simulink model "EV_PV_Charging"  (R2025a)
settings: Solver=ode3  StartTime=0.0  StopTime=1  RelTol=1e-3
PreLoadFcn:
  | %% Parameter file: OBC_4_data.m
  | 
  | %% Model Parameters
  | Ts_Power= 50e-9;        % SPS Model sample time (s)
  | Co=150e-6;              % Output filter (F)
  | Ron_FET=50e-3;          % FET resistance (ohms)
  | Ron_Diode=50e-3;        % FET resistance (ohms)
  | Vf=0.6;                 % Diode forward voltage (V)
  | %
  | %% PFC Data
  | Vnom_ac= 240;           % Nominal Ac voltage (V)
  | Fnom= 60;               % System frequency (Hz)
  | L_PFC= 600e-6;          % PFC Inductance (H)
  | RL_PFC= 20e-3;          % Inductance resistance (Ohm)
  | C_PFC= 2600e-6;         % Capacitance (F)
  | 
  | %% PFC Control System Parameters
  | Ts_Control= 10e-6;      % Control system time (s)
  | Fsw= 100e3;             % PWM Switching frequency (Hz)
  | DT_PFC=400e-9;
  | %
  | % Current Regulator (PR):
  | Kp_I= 0.06;             % Proportional gain
  | Kr_I= 2.5;              % Resonant gain
  | Zeta_I=0.2;             % Damping coefficient
  | Fr_I=Fnom*2;            % Resonant frequency (Hz)
  | %
  | % Voltage Regulator (PI):
  | Kp_V= 0.25;             % Proportional gain
  | Ki_V= 80;               % Integral gain
  | Limit_V= 100;           % Output limit
  | %
  | %% LLC Data
  | Vdc_in=400;             % DC input voltage (V)
  | Vo_nom=400;             % DC nominal output voltage (V)
  | Po_nom=7.2e3;           % Nominal output power (W)
  | Lr=25e-6;               % Transformer leakage inductance (Resonant inductance in Henry)
  | Lm=150e-6;              % Magnetization inductance (H)
  | Cr=75e-9;               % Resonant capacitor (F)
  | Np=10; Ns=12; N=Np/Ns;  % Transformer ratio
  | %
  | %% LLC Control System Parameters
  | DT_LLC=400e-9;
  | Ts_Control=10e-6;
  | % Voltage Regulator (PI):
  | Kp_LLC= 100/4;          % Proportional gain
  | Ki_LLC= 150e3;          % Integral gain
  | fs_LCC_min= 120e3;      % Minimum switching frequency (Hz)
  | fs_LCC_max= 300e3;      % Maximum switching frequency (Hz)
  | Vref_LCC_min= 275;      % Minimum voltage setpoint (V)
  | Vref_LCC_max= 450;      % Maximum voltage setpoint (V)
  | %
  | %%
  | % Resonant tank data
  | Ro=Vo_nom^2/Po_nom      % LLC output load (Ohm)
  | Rac=(8/pi^2)*N^2*Ro     % Equivalent pprimary AC resistance (Ohm)
  | Q=sqrt(Lr/Cr)/Rac       % Quality factor
  | fr=1/(2*pi*sqrt(Lr*Cr)) % Resonant frequency (Hz)
  | m=(Lr+Lm)/Lr            % Ratio of total primary reactance to resonant inductance (Lr)
  | %%
InitFcn:
  | %% Parameter file: OBC_4_data.m
  | 
  | %% Model Parameters
  | Ts_Power= 50e-9;        % SPS Model sample time (s)
  | Co=150e-6;              % Output filter (F)
  | Ron_FET=50e-3;          % FET resistance (ohms)
  | Ron_Diode=50e-3;        % FET resistance (ohms)
  | Vf=0.6;                 % Diode forward voltage (V)
  | %
  | %% PFC Data
  | Vnom_ac= 240;           % Nominal Ac voltage (V)
  | Fnom= 60;               % System frequency (Hz)
  | L_PFC= 600e-6;          % PFC Inductance (H)
  | RL_PFC= 20e-3;          % Inductance resistance (Ohm)
  | C_PFC= 2600e-6;         % Capacitance (F)
  | 
  | %% PFC Control System Parameters
  | Ts_Control= 10e-6;      % Control system time (s)
  | Fsw= 100e3;             % PWM Switching frequency (Hz)
  | DT_PFC=400e-9;
  | %
  | % Current Regulator (PR):
  | Kp_I= 0.06;             % Proportional gain
  | Kr_I= 2.5;              % Resonant gain
  | Zeta_I=0.2;             % Damping coefficient
  | Fr_I=Fnom*2;            % Resonant frequency (Hz)
  | %
  | % Voltage Regulator (PI):
  | Kp_V= 0.25;             % Proportional gain
  | Ki_V= 80;               % Integral gain
  | Limit_V= 100;           % Output limit
  | %
  | %% LLC Data
  | Vdc_in=400;             % DC input voltage (V)
  | Vo_nom=400;             % DC nominal output voltage (V)
  | Po_nom=7.2e3;           % Nominal output power (W)
  | Lr=25e-6;               % Transformer leakage inductance (Resonant inductance in Henry)
  | Lm=150e-6;              % Magnetization inductance (H)
  | Cr=75e-9;               % Resonant capacitor (F)
  | Np=10; Ns=12; N=Np/Ns;  % Transformer ratio
  | %
  | %% LLC Control System Parameters
  | DT_LLC=400e-9;
  | Ts_Control=10e-6;
  | % Voltage Regulator (PI):
  | Kp_LLC= 100/4;          % Proportional gain
  | Ki_LLC= 150e3;          % Integral gain
  | fs_LCC_min= 120e3;      % Minimum switching frequency (Hz)
  | fs_LCC_max= 300e3;      % Maximum switching frequency (Hz)
  | Vref_LCC_min= 275;      % Minimum voltage setpoint (V)
  | Vref_LCC_max= 450;      % Maximum voltage setpoint (V)
  | %
  | %%
  | % Resonant tank data
  | Ro=Vo_nom^2/Po_nom      % LLC output load (Ohm)
  | Rac=(8/pi^2)*N^2*Ro     % Equivalent pprimary AC resistance (Ohm)
  | Q=sqrt(Lr/Cr)/Rac       % Quality factor
  | fr=1/(2*pi*sqrt(Lr*Cr)) % Resonant frequency (Hz)
  | m=(Lr+Lm)/Lr            % Ratio of total primary reactance to resonant inductance (Lr)
  | %%
undefined symbols (not defined in the file or in its folder): D1, Delta, DiscIntNeverNeededParam
libraries: spsSeriesRLCBranchLib x11, spsDiodeLib x7, spsMeanLib x6, MyLibrary x6, spsCurrentMeasurementLib x5, spsVoltageMeasurementLib x5, spsFourierLib x4, spsThreePhaseTransformerTwoWindingsLib x3, spsOnDelayLib x3, spsDistributedParametersLineLib x2, spsThreePhaseParallelRLCLoadLib x2, spsPWMGeneratorDCDCLib x2
(part 2 of 4)

== system EV_PV_Charging/600V Utlity Grid ==
  120 kV / 25 kV 47 MVA : spsThreePhaseTransformerTwoWindingsLib/Three-Phase Transformer (Two Windings)  Winding1Connection=Yg  Winding2Connection=Delta (D1)  CoreType=Three single-phase transformers  SetSaturation=off  Hysteresis=off  DataFile='basic_model'  SetInitialFlux=off  Measurements=None  UNITS=pu  NominalPower=[47e6 60 ]  Winding1="[ 120e3  0.08/30   0.08 ]"  Winding2="[ 25e3  0.08/30  0.08]"  Rm=500  Lm=500  L0=0.5  Saturation="[ 0,0  ;  0.005,1.2  ;  1.0,1.4 ]"  InitialFluxes=[ 0.8 , -0.8 , 0.7 ]  BreakLoop=off  DiscreteSolver=Trapezoidal iterative  DataType=off  TransfoNumber=0
  120kV 2500MVA : spsThreePhaseSourceLib/Three-Phase Source  InternalConnection=Yg  VoltagePhases=off  Voltage=120e3  PhaseAngle=0  Voltage_phases=[25e3 25e3 25e3]/sqrt(3)  PhaseAngles_phases=[0 -120 +120]  Frequency=60  NonIdealSource=on  SpecifyImpedance=on  Resistance=0.8929  Inductance=16.58e-3  ShortCircuitLevel=2500e6  BaseVoltage=120e3  XRratio=7  BusType=swing  Pref=0  Qref=0  Prefabc=[10e3, 10e3, 10e3]  Qrefabc=[0, 0, 0]  Qmin=-inf  Qmax=inf
  14-km Feeder : spsDistributedParametersLineLib/Distributed Parameters Line  Phases=3  Length=14  Frequency=60  Resistance=[0.1153 0.413]  Inductance=[1.05e-3 3.32e-3]  Capacitance=[11.33e-009 5.01e-009]  x1=[-5.71e-05 -1.91453846184522e-09 0 0;-5.705e-05 -1.91458738877014e-09 0 0;-5.7e-05 -1.9146363150148e-09 0 0;-5.695e-05 -1.91468524057917e-09 0 0;-5.69e-05 -1.91473416546325e-09 0 0;-5.685e-05 -1.91478308966701e-09 0 0;-5.68e-05 -1.91483201319044e-09 0 0;-5.675e-05 -1.91488093603352e-09 0 0;-5.67e-05 -1.91492985819623e-09 0 0;-5.665e-05 -1.91497877967855e-09 0 0;-5.66e-05 -1.91502770048047e-09 0 0;-5.655e-05 -1.91507662060197e-09 0 0;-5.65e-05 -1.91512554004303e-09 0 0;-5.645e-05 -1.91517445880364e-09 0 0;-5.64e-05 -1.91522337688377e-09 0 0;-5.635e-05 -1.91527229428342e-09 0 0;-5.63e-05 -1.91532121100256e-09 0 0;-5.625e-05 -1.91537012704117e-09 0 0;-5.62e-05 -1.91541904239924e-09 0 0;-5.615e-05 -1.91546795707675e-09 0 0;-5.61e-05 -1.91551687107368e-09 0 0;-5.605e-05 -1.91556578439002e-09 0 0;-5.6e-05 -1.91561469702575e-09 0 0;-5.595e-05 -1.91566360898085e-09 0 0;-5.59e-05 -1.91571252025531e-09 0 0;-5.585e-05 -1.9157614308491e-09 0 0;-5.58e-05 -1.9158103407622e-09 0 0;-5.575e-05 -1.91585924999461e-09 0 0;-5.57e-05 -1.91590815854631e-09 0 0;-5.565e-05 -1.91595706641727e-09 0 0;-5.56e-05 -1.91600597360748e-09 0 0;-5.555e-05 -1.91605488011692e-09 0 0;-5.55e-05 -1.91610378594558e-09 0 0;-5.545e-05 -1.91615269109344e-09 0 0;-5.54e-05 -1.91620159556047e-09 0 0;-5.535e-05 -1.91625049934667e-09 0 0;-5.53e-05 -1.91629940245201e-09 0 0;-5.525e-05 -1.91634830487648e-09 0 0;-5.52e-05 -1.91639720662006e-09 0 0;-5.515e-05 -1.91644610768273e-09 0 0;-5.51e-05 -1.91649500806448e-09 0 0;-5.505e-05 -1.91654390776529e-09 0 0;-5.5e-05 -1.91659280678514e-09 0 0;-5.495e-05 -1.91664170512401e-09 0 0;-5.49e-05 -1.91669060278189e-09 0 0;-5.485e-05 -1.91673949975876e-09 0 0;-5.48e-05 -1.91678839605459e-09 0 0;-5.475e-05 -1.91683729166939e-09 0 0;-5.47e-05 -1.91688618660312e-09 0 0;-5.465e-05 -1.91693508085576e-09 0 0;-5.46e-05 -1.91698397442731e-09 0 0;-5.455e-05 -1.91703286731775e-09 0 0;-5.45e-05 -1.91708175952705e-09 0 0;-5.445e-05 -1.9171306510552e-09 0 0;-5.44e-05 -1.91717954190219e-09 0 0;-5.435e-05 -1.91722843206799e-09 0 0;-5.43e-05 -1.91727732155258e-09 0 0;-5.425e-05 -1.91732621035596e-09 0 0;-5.42e-05 -1.9173750984781e-09 0 0;-5.415e-05 -1.91742398591899e-09 0 0;-5.41e-05 -1.9174728726786e-09 0 0;-5.405e-05 -1.91752175875693e-09 0 0;-5.4e-05 -1.91757064415394e-09 0 0;-5.395e-05 -1.91761952886964e-09 0 0;-5.39e-05 -1.91766841290399e-09 0 0;-5.385e-05 -1.91771729625699e-09 0 0;-5.38e-05 -1.91776617892861e-09 0 0;-5.375e-05 -1.91781506091883e-09 0 0;-5.37e-05 -1.91786394222765e-09 0 0;-5.365e-05 -1.91791282285503e-09 0 0;-5.36e-05 -1.91796170280097e-09 0 0;-5.355e-05 -1.91801058206545e-09 0 0;-5.35e-05 -1.91805946064845e-09 0 0;-5.345e-05 -1.91810833854995e-09 0 0;-5.34e-05 -1.91815721576993e-09 0 0;-5.335e-05 -1.91820609230839e-09 0 0;-5.33e-05 -1.91825496816529e-09 0 0;-5.325e-05 -1.91830384334063e-09 0 0;-5.32e-05 -1.91835271783438e-09 0 0;-5.315e-05 -1.91840159164653e-09 0 0;-5.31e-05 -1.91845046477706e-09 0 0;-5.305e-05 -1.91849933722596e-09 0 0;-5.3e-05 -1.9185482089932e-09 0 0;-5.295e-05 -1.91859708007877e-09 0 0;-5.29e-05 -1.91864595048265e-09 0 0;-5.285e-05 -1.91869482020482e-09 0 0;-5.28e-05 -1.91874368924527e-09 0 0;-5.275e-05 -1.91879255760398e-09 0 0;-5.27e-05 -1.91884142528094e-09 0 0;-5.265e-05 -1.91889029227611e-09 0 0;-5.26e-05 -1.9189391585895e-09 0 0;-5.255e-05 -1.91898802422107e-09 0 0;-5.25e-05 -1.91903688917082e-09 0 0;-5.245e-05 -1.91908575343872e-09 0 0;-5.24e-05 -1.91913461702476e-09 0 0;-5.235e-05 -1.91918347992892e-09 0 0;-5.23e-05 -1.91923234215119e-09 0 0;-5.225e-05 -1.91928120369154e-09 0 0;-5.22e-05 -1.91933006454995e-09 0 0;-5.215e-05 -1.91937892472642e-09 0 0;-5.21e-05 -1.91942778422092e-09 0 0;-5.205e-05 -1.91947664303344e-09 0 0;-5.2e-05 -1.91952550116396e-09 0 0;-5.195e-05 -1.91957435861246e-09 0 0;-5.19e-05 -1.91962321537892e-09 0 0;-5.185e-05 -1.91967207146333e-09 0 0;-5.18e-05 -1.91972092686567e-09 0 0;-5.175e-05 -1.91976978158592e-09 0 0;-5.17e-05 -1.91981863562407e-09 0 0;-5.165e-05 -1.91986748898009e-09 0 ...(+67941 chars)]  x2=[-5.71e-05 -2.09426061623554e-09 0 0;-5.705e-05 -2.09430829998972e-09 0 0;-5.7e-05 -2.09435598299977e-09 0 0;-5.695e-05 -2.09440366526568e-09 0 0;-5.69e-05 -2.09445134678745e-09 0 0;-5.685e-05 -2.09449902756504e-09 0 0;-5.68e-05 -2.09454670759844e-09 0 0;-5.675e-05 -2.09459438688764e-09 0 0;-5.67e-05 -2.09464206543262e-09 0 0;-5.665e-05 -2.09468974323336e-09 0 0;-5.66e-05 -2.09473742028984e-09 0 0;-5.655e-05 -2.09478509660205e-09 0 0;-5.65e-05 -2.09483277216998e-09 0 0;-5.645e-05 -2.09488044699359e-09 0 0;-5.64e-05 -2.09492812107289e-09 0 0;-5.635e-05 -2.09497579440784e-09 0 0;-5.63e-05 -2.09502346699844e-09 0 0;-5.625e-05 -2.09507113884466e-09 0 0;-5.62e-05 -2.09511880994649e-09 0 0;-5.615e-05 -2.09516648030391e-09 0 0;-5.61e-05 -2.09521414991691e-09 0 0;-5.605e-05 -2.09526181878547e-09 0 0;-5.6e-05 -2.09530948690957e-09 0 0;-5.595e-05 -2.09535715428919e-09 0 0;-5.59e-05 -2.09540482092432e-09 0 0;-5.585e-05 -2.09545248681495e-09 0 0;-5.58e-05 -2.09550015196104e-09 0 0;-5.575e-05 -2.09554781636259e-09 0 0;-5.57e-05 -2.09559548001959e-09 0 0;-5.565e-05 -2.095643142932e-09 0 0;-5.56e-05 -2.09569080509982e-09 0 0;-5.555e-05 -2.09573846652303e-09 0 0;-5.55e-05 -2.09578612720161e-09 0 0;-5.545e-05 -2.09583378713555e-09 0 0;-5.54e-05 -2.09588144632482e-09 0 0;-5.535e-05 -2.09592910476942e-09 0 0;-5.53e-05 -2.09597676246932e-09 0 0;-5.525e-05 -2.09602441942451e-09 0 0;-5.52e-05 -2.09607207563497e-09 0 0;-5.515e-05 -2.09611973110068e-09 0 0;-5.51e-05 -2.09616738582163e-09 0 0;-5.505e-05 -2.09621503979779e-09 0 0;-5.5e-05 -2.09626269302917e-09 0 0;-5.495e-05 -2.09631034551572e-09 0 0;-5.49e-05 -2.09635799725745e-09 0 0;-5.485e-05 -2.09640564825433e-09 0 0;-5.48e-05 -2.09645329850634e-09 0 0;-5.475e-05 -2.09650094801347e-09 0 0;-5.47e-05 -2.0965485967757e-09 0 0;-5.465e-05 -2.09659624479302e-09 0 0;-5.46e-05 -2.0966438920654e-09 0 0;-5.455e-05 -2.09669153859283e-09 0 0;-5.45e-05 -2.0967391843753e-09 0 0;-5.445e-05 -2.09678682941278e-09 0 0;-5.44e-05 -2.09683447370527e-09 0 0;-5.435e-05 -2.09688211725273e-09 0 0;-5.43e-05 -2.09692976005516e-09 0 0;-5.425e-05 -2.09697740211254e-09 0 0;-5.42e-05 -2.09702504342485e-09 0 0;-5.415e-05 -2.09707268399208e-09 0 0;-5.41e-05 -2.09712032381421e-09 0 0;-5.405e-05 -2.09716796289121e-09 0 0;-5.4e-05 -2.09721560122308e-09 0 0;-5.395e-05 -2.0972632388098e-09 0 0;-5.39e-05 -2.09731087565135e-09 0 0;-5.385e-05 -2.09735851174771e-09 0 0;-5.38e-05 -2.09740614709887e-09 0 0;-5.375e-05 -2.0974537817048e-09 0 0;-5.37e-05 -2.0975014155655e-09 0 0;-5.365e-05 -2.09754904868095e-09 0 0;-5.36e-05 -2.09759668105112e-09 0 0;-5.355e-05 -2.09764431267601e-09 0 0;-5.35e-05 -2.09769194355559e-09 0 0;-5.345e-05 -2.09773957368985e-09 0 0;-5.34e-05 -2.09778720307877e-09 0 0;-5.335e-05 -2.09783483172233e-09 0 0;-5.33e-05 -2.09788245962052e-09 0 0;-5.325e-05 -2.09793008677332e-09 0 0;-5.32e-05 -2.09797771318072e-09 0 0;-5.315e-05 -2.09802533884269e-09 0 0;-5.31e-05 -2.09807296375922e-09 0 0;-5.305e-05 -2.09812058793029e-09 0 0;-5.3e-05 -2.09816821135589e-09 0 0;-5.295e-05 -2.098215834036e-09 0 0;-5.29e-05 -2.0982634559706e-09 0 0;-5.285e-05 -2.09831107715967e-09 0 0;-5.28e-05 -2.0983586976032e-09 0 0;-5.275e-05 -2.09840631730118e-09 0 0;-5.27e-05 -2.09845393625358e-09 0 0;-5.265e-05 -2.09850155446038e-09 0 0;-5.26e-05 -2.09854917192158e-09 0 0;-5.255e-05 -2.09859678863714e-09 0 0;-5.25e-05 -2.09864440460707e-09 0 0;-5.245e-05 -2.09869201983133e-09 0 0;-5.24e-05 -2.09873963430992e-09 0 0;-5.235e-05 -2.09878724804281e-09 0 0;-5.23e-05 -2.09883486103e-09 0 0;-5.225e-05 -2.09888247327145e-09 0 0;-5.22e-05 -2.09893008476716e-09 0 0;-5.215e-05 -2.0989776955171e-09 0 0;-5.21e-05 -2.09902530552127e-09 0 0;-5.205e-05 -2.09907291477964e-09 0 0;-5.2e-05 -2.0991205232922e-09 0 0;-5.195e-05 -2.09916813105893e-09 0 0;-5.19e-05 -2.09921573807982e-09 0 0;-5.185e-05 -2.09926334435484e-09 0 0;-5.18e-05 -2.09931094988398e-09 0 0;-5.175e-05 -2.09935855466722e-09 0 0;-5.17e-05 -2.09940615870455e-09 0 0;-5.165e-05 -2.09945376199594e-09 0 0 ...(+67971 chars)]  x3=[-5.71e-05 -8.597316094106e-12 0 0;-5.705e-05 -8.59751457746718e-12 0 0;-5.7e-05 -8.59771305777361e-12 0 0;-5.695e-05 -8.59791153502522e-12 0 0;-5.69e-05 -8.59811000922194e-12 0 0;-5.685e-05 -8.59830848036371e-12 0 0;-5.68e-05 -8.59850694845045e-12 0 0;-5.675e-05 -8.59870541348209e-12 0 0;-5.67e-05 -8.59890387545856e-12 0 0;-5.665e-05 -8.59910233437979e-12 0 0;-5.66e-05 -8.59930079024571e-12 0 0;-5.655e-05 -8.59949924305624e-12 0 0;-5.65e-05 -8.59969769281133e-12 0 0;-5.645e-05 -8.59989613951089e-12 0 0;-5.64e-05 -8.60009458315487e-12 0 0;-5.635e-05 -8.60029302374318e-12 0 0;-5.63e-05 -8.60049146127575e-12 0 0;-5.625e-05 -8.60068989575252e-12 0 0;-5.62e-05 -8.60088832717341e-12 0 0;-5.615e-05 -8.60108675553837e-12 0 0;-5.61e-05 -8.6012851808473e-12 0 0;-5.605e-05 -8.60148360310015e-12 0 0;-5.6e-05 -8.60168202229684e-12 0 0;-5.595e-05 -8.60188043843731e-12 0 0;-5.59e-05 -8.60207885152148e-12 0 0;-5.585e-05 -8.60227726154928e-12 0 0;-5.58e-05 -8.60247566852064e-12 0 0;-5.575e-05 -8.60267407243549e-12 0 0;-5.57e-05 -8.60287247329376e-12 0 0;-5.565e-05 -8.60307087109538e-12 0 0;-5.56e-05 -8.60326926584028e-12 0 0;-5.555e-05 -8.60346765752839e-12 0 0;-5.55e-05 -8.60366604615964e-12 0 0;-5.545e-05 -8.60386443173396e-12 0 0;-5.54e-05 -8.60406281425127e-12 0 0;-5.535e-05 -8.60426119371152e-12 0 0;-5.53e-05 -8.60445957011461e-12 0 0;-5.525e-05 -8.60465794346049e-12 0 0;-5.52e-05 -8.60485631374909e-12 0 0;-5.515e-05 -8.60505468098034e-12 0 0;-5.51e-05 -8.60525304515416e-12 0 0;-5.505e-05 -8.60545140627048e-12 0 0;-5.5e-05 -8.60564976432923e-12 0 0;-5.495e-05 -8.60584811933035e-12 0 0;-5.49e-05 -8.60604647127377e-12 0 0;-5.485e-05 -8.6062448201594e-12 0 0;-5.48e-05 -8.60644316598719e-12 0 0;-5.475e-05 -8.60664150875705e-12 0 0;-5.47e-05 -8.60683984846893e-12 0 0;-5.465e-05 -8.60703818512275e-12 0 0;-5.46e-05 -8.60723651871843e-12 0 0;-5.455e-05 -8.60743484925592e-12 0 0;-5.45e-05 -8.60763317673514e-12 0 0;-5.445e-05 -8.60783150115601e-12 0 0;-5.44e-05 -8.60802982251847e-12 0 0;-5.435e-05 -8.60822814082245e-12 0 0;-5.43e-05 -8.60842645606788e-12 0 0;-5.425e-05 -8.60862476825468e-12 0 0;-5.42e-05 -8.60882307738279e-12 0 0;-5.415e-05 -8.60902138345213e-12 0 0;-5.41e-05 -8.60921968646264e-12 0 0;-5.405e-05 -8.60941798641425e-12 0 0;-5.4e-05 -8.60961628330688e-12 0 0;-5.395e-05 -8.60981457714046e-12 0 0;-5.39e-05 -8.61001286791492e-12 0 0;-5.385e-05 -8.6102111556302e-12 0 0;-5.38e-05 -8.61040944028622e-12 0 0;-5.375e-05 -8.61060772188291e-12 0 0;-5.37e-05 -8.61080600042021e-12 0 0;-5.365e-05 -8.61100427589803e-12 0 0;-5.36e-05 -8.61120254831632e-12 0 0;-5.355e-05 -8.61140081767499e-12 0 0;-5.35e-05 -8.61159908397399e-12 0 0;-5.345e-05 -8.61179734721323e-12 0 0;-5.34e-05 -8.61199560739266e-12 0 0;-5.335e-05 -8.61219386451219e-12 0 0;-5.33e-05 -8.61239211857176e-12 0 0;-5.325e-05 -8.6125903695713e-12 0 0;-5.32e-05 -8.61278861751073e-12 0 0;-5.315e-05 -8.61298686238999e-12 0 0;-5.31e-05 -8.61318510420901e-12 0 0;-5.305e-05 -8.61338334296771e-12 0 0;-5.3e-05 -8.61358157866603e-12 0 0;-5.295e-05 -8.6137798113039e-12 0 0;-5.29e-05 -8.61397804088123e-12 0 0;-5.285e-05 -8.61417626739797e-12 0 0;-5.28e-05 -8.61437449085405e-12 0 0;-5.275e-05 -8.61457271124939e-12 0 0;-5.27e-05 -8.61477092858392e-12 0 0;-5.265e-05 -8.61496914285757e-12 0 0;-5.26e-05 -8.61516735407028e-12 0 0;-5.255e-05 -8.61536556222196e-12 0 0;-5.25e-05 -8.61556376731256e-12 0 0;-5.245e-05 -8.615761969342e-12 0 0;-5.24e-05 -8.61596016831021e-12 0 0;-5.235e-05 -8.61615836421711e-12 0 0;-5.23e-05 -8.61635655706265e-12 0 0;-5.225e-05 -8.61655474684675e-12 0 0;-5.22e-05 -8.61675293356933e-12 0 0;-5.215e-05 -8.61695111723033e-12 0 0;-5.21e-05 -8.61714929782968e-12 0 0;-5.205e-05 -8.61734747536731e-12 0 0;-5.2e-05 -8.61754564984315e-12 0 0;-5.195e-05 -8.61774382125712e-12 0 0;-5.19e-05 -8.61794198960916e-12 0 0;-5.185e-05 -8.61814015489919e-12 0 0;-5.18e-05 -8.61833831712715e-12 0 0;-5.175e-05 -8.61853647629296e-12 0 0;-5.17e-05 -8.61873463239655e-12 0 0;-5.165e-05 -8.61893278543787e-12 0 ...(+67945 chars)]  x4=[-5.71e-05 4.32288377505827e-12 0 0;-5.705e-05 4.32297924503688e-12 0 0;-5.7e-05 4.3230747134795e-12 0 0;-5.695e-05 4.32317018038611e-12 0 0;-5.69e-05 4.32326564575667e-12 0 0;-5.685e-05 4.32336110959115e-12 0 0;-5.68e-05 4.32345657188952e-12 0 0;-5.675e-05 4.32355203265173e-12 0 0;-5.67e-05 4.32364749187777e-12 0 0;-5.665e-05 4.32374294956758e-12 0 0;-5.66e-05 4.32383840572115e-12 0 0;-5.655e-05 4.32393386033843e-12 0 0;-5.65e-05 4.32402931341939e-12 0 0;-5.645e-05 4.324124764964e-12 0 0;-5.64e-05 4.32422021497223e-12 0 0;-5.635e-05 4.32431566344403e-12 0 0;-5.63e-05 4.32441111037938e-12 0 0;-5.625e-05 4.32450655577824e-12 0 0;-5.62e-05 4.32460199964058e-12 0 0;-5.615e-05 4.32469744196636e-12 0 0;-5.61e-05 4.32479288275556e-12 0 0;-5.605e-05 4.32488832200813e-12 0 0;-5.6e-05 4.32498375972404e-12 0 0;-5.595e-05 4.32507919590326e-12 0 0;-5.59e-05 4.32517463054575e-12 0 0;-5.585e-05 4.32527006365149e-12 0 0;-5.58e-05 4.32536549522043e-12 0 0;-5.575e-05 4.32546092525254e-12 0 0;-5.57e-05 4.3255563537478e-12 0 0;-5.565e-05 4.32565178070616e-12 0 0;-5.56e-05 4.32574720612758e-12 0 0;-5.555e-05 4.32584263001205e-12 0 0;-5.55e-05 4.32593805235952e-12 0 0;-5.545e-05 4.32603347316996e-12 0 0;-5.54e-05 4.32612889244333e-12 0 0;-5.535e-05 4.32622431017961e-12 0 0;-5.53e-05 4.32631972637875e-12 0 0;-5.525e-05 4.32641514104073e-12 0 0;-5.52e-05 4.32651055416551e-12 0 0;-5.515e-05 4.32660596575305e-12 0 0;-5.51e-05 4.32670137580332e-12 0 0;-5.505e-05 4.3267967843163e-12 0 0;-5.5e-05 4.32689219129193e-12 0 0;-5.495e-05 4.3269875967302e-12 0 0;-5.49e-05 4.32708300063106e-12 0 0;-5.485e-05 4.32717840299449e-12 0 0;-5.48e-05 4.32727380382044e-12 0 0;-5.475e-05 4.32736920310889e-12 0 0;-5.47e-05 4.3274646008598e-12 0 0;-5.465e-05 4.32755999707314e-12 0 0;-5.46e-05 4.32765539174887e-12 0 0;-5.455e-05 4.32775078488696e-12 0 0;-5.45e-05 4.32784617648737e-12 0 0;-5.445e-05 4.32794156655008e-12 0 0;-5.44e-05 4.32803695507504e-12 0 0;-5.435e-05 4.32813234206223e-12 0 0;-5.43e-05 4.3282277275116e-12 0 0;-5.425e-05 4.32832311142314e-12 0 0;-5.42e-05 4.32841849379679e-12 0 0;-5.415e-05 4.32851387463253e-12 0 0;-5.41e-05 4.32860925393033e-12 0 0;-5.405e-05 4.32870463169015e-12 0 0;-5.4e-05 4.32880000791195e-12 0 0;-5.395e-05 4.3288953825957e-12 0 0;-5.39e-05 4.32899075574138e-12 0 0;-5.385e-05 4.32908612734894e-12 0 0;-5.38e-05 4.32918149741834e-12 0 0;-5.375e-05 4.32927686594957e-12 0 0;-5.37e-05 4.32937223294258e-12 0 0;-5.365e-05 4.32946759839734e-12 0 0;-5.36e-05 4.32956296231381e-12 0 0;-5.355e-05 4.32965832469196e-12 0 0;-5.35e-05 4.32975368553177e-12 0 0;-5.345e-05 4.32984904483318e-12 0 0;-5.34e-05 4.32994440259618e-12 0 0;-5.335e-05 4.33003975882072e-12 0 0;-5.33e-05 4.33013511350677e-12 0 0;-5.325e-05 4.3302304666543e-12 0 0;-5.32e-05 4.33032581826328e-12 0 0;-5.315e-05 4.33042116833366e-12 0 0;-5.31e-05 4.33051651686543e-12 0 0;-5.305e-05 4.33061186385853e-12 0 0;-5.3e-05 4.33070720931294e-12 0 0;-5.295e-05 4.33080255322863e-12 0 0;-5.29e-05 4.33089789560556e-12 0 0;-5.285e-05 4.3309932364437e-12 0 0;-5.28e-05 4.33108857574301e-12 0 0;-5.275e-05 4.33118391350345e-12 0 0;-5.27e-05 4.33127924972501e-12 0 0;-5.265e-05 4.33137458440763e-12 0 0;-5.26e-05 4.3314699175513e-12 0 0;-5.255e-05 4.33156524915596e-12 0 0;-5.25e-05 4.3316605792216e-12 0 0;-5.245e-05 4.33175590774817e-12 0 0;-5.24e-05 4.33185123473565e-12 0 0;-5.235e-05 4.33194656018399e-12 0 0;-5.23e-05 4.33204188409317e-12 0 0;-5.225e-05 4.33213720646315e-12 0 0;-5.22e-05 4.33223252729389e-12 0 0;-5.215e-05 4.33232784658537e-12 0 0;-5.21e-05 4.33242316433755e-12 0 0;-5.205e-05 4.33251848055039e-12 0 0;-5.2e-05 4.33261379522386e-12 0 0;-5.195e-05 4.33270910835793e-12 0 0;-5.19e-05 4.33280441995257e-12 0 0;-5.185e-05 4.33289973000773e-12 0 0;-5.18e-05 4.33299503852339e-12 0 0;-5.175e-05 4.33309034549951e-12 0 0;-5.17e-05 4.33318565093606e-12 0 0;-5.165e-05 4.333280954833e-12 0 0;-5.16e-05 4.33337625719031e-12 0 0;-5.155e-05 4.33347155800794e-12 0 0;-5.15e-05 4.33356685728586e-12 0 0 ...(+66820 chars)]  x5=5.70973484498186e-05  V1=[0 0 0 2.868e-09 2.436e+04 2.436e+04;0 0 0 377 377 377;1.571 1.571 1.571 -0.5389 -0.156 -1.727]  V2=[0 0 0 2.996e-09 2.448e+04 2.448e+04;0 0 0 377 377 377;1.571 1.571 1.571 -0.5232 -0.1382 -1.709]  I1=[0 0 0 1.022e-11 157.5 157.5;0 0 0 377 377 377;1.571 1.571 1.571 -1.198 -0.1498 -1.721]  I2=[0 0 0 6.231e-12 2.544 2.544;0 0 0 377 377 377;1.571 1.571 1.571 1.184 -0.5617 -2.133]  nHarmo=2  Measurements=None  Decoupling=off  VsMag0=0  VrMag0=0  VsAngle0=0  VrAngle0=0  IsMag0=0  IrMag0=0  IsAngle0=0  IrAngle0=0
  2-MW Load : spsThreePhaseParallelRLCLoadLib/Three-Phase Parallel RLC Load  LConnTagsString=A|B|C  Configuration=Y (grounded)  NominalVoltage=25e3  Vabc=[1e3 1e3 1e3]  Vabcp=[1e3 1e3 1e3]  NominalFrequency=60  UnbalancedPower=off  ActivePower=2e6  InductivePower=0  CapacitivePower=0  Pabc=[10e3 9e3 11e3]  QLabc=[100 90 110]  QCabc=[100 90 110]  Pabcp=[10e3 9e3 11e3]  QLabcp=[100 90 110]  QCabcp=[100 90 110]  Measurements=None  LoadType=constant Z
  "3.3ohms " : spsSeriesRLCBranchLib/Series RLC Branch  LConnTagsString=__new0  RConnTagsString=__new0  BranchType=R  Resistance=3.3  Inductance=[]  SetiL0=off  InitialCurrent=0  Capacitance=[]  Setx0=off  InitialVoltage=0  Measurements=None
  30-MW 2-Mvar Load : spsThreePhaseParallelRLCLoadLib/Three-Phase Parallel RLC Load  LConnTagsString=A|B|C  Configuration=Y (grounded)  NominalVoltage=25e3  Vabc=[1e3 1e3 1e3]  Vabcp=[1e3 1e3 1e3]  NominalFrequency=60  UnbalancedPower=off  ActivePower=30e6  InductivePower=2e6  CapacitivePower=0  Pabc=[10e3 9e3 11e3]  QLabc=[100 90 110]  QCabc=[100 90 110]  Pabcp=[10e3 9e3 11e3]  QLabcp=[100 90 110]  QCabcp=[100 90 110]  Measurements=None  LoadType=constant Z
  5-km Feeder : spsDistributedParametersLineLib/Distributed Parameters Line  Phases=3  Length=5  Frequency=60  Resistance=[0.1153 0.413]  Inductance=[1.05e-3 3.32e-3]  Capacitance=[11.33e-009 5.01e-009]  x1=[-2.04e-05 -1.94923131916929e-09 0 0;-2.035e-05 -1.9492800505635e-09 0 0;-2.03e-05 -1.94932878126512e-09 0 0;-2.025e-05 -1.94937751127413e-09 0 0;-2.02e-05 -1.94942624059052e-09 0 0;-2.015e-05 -1.94947496921427e-09 0 0;-2.01e-05 -1.94952369714535e-09 0 0;-2.005e-05 -1.94957242438376e-09 0 0;-2e-05 -1.94962115092947e-09 0 0;-1.995e-05 -1.94966987678248e-09 0 0;-1.99e-05 -1.94971860194275e-09 0 0;-1.985e-05 -1.94976732641028e-09 0 0;-1.98e-05 -1.94981605018504e-09 0 0;-1.975e-05 -1.94986477326702e-09 0 0;-1.97e-05 -1.94991349565621e-09 0 0;-1.965e-05 -1.94996221735258e-09 0 0;-1.96e-05 -1.95001093835611e-09 0 0;-1.955e-05 -1.9500596586668e-09 0 0;-1.95e-05 -1.95010837828462e-09 0 0;-1.945e-05 -1.95015709720955e-09 0 0;-1.94e-05 -1.95020581544158e-09 0 0;-1.935e-05 -1.95025453298069e-09 0 0;-1.93e-05 -1.95030324982687e-09 0 0;-1.925e-05 -1.95035196598009e-09 0 0;-1.92e-05 -1.95040068144034e-09 0 0;-1.915e-05 -1.95044939620761e-09 0 0;-1.91e-05 -1.95049811028186e-09 0 0;-1.905e-05 -1.95054682366309e-09 0 0;-1.9e-05 -1.95059553635129e-09 0 0;-1.895e-05 -1.95064424834642e-09 0 0;-1.89e-05 -1.95069295964848e-09 0 0;-1.885e-05 -1.95074167025745e-09 0 0;-1.88e-05 -1.9507903801733e-09 0 0;-1.875e-05 -1.95083908939603e-09 0 0;-1.87e-05 -1.95088779792562e-09 0 0;-1.865e-05 -1.95093650576204e-09 0 0;-1.86e-05 -1.95098521290529e-09 0 0;-1.855e-05 -1.95103391935534e-09 0 0;-1.85e-05 -1.95108262511217e-09 0 0;-1.845e-05 -1.95113133017578e-09 0 0;-1.84e-05 -1.95118003454613e-09 0 0;-1.835e-05 -1.95122873822323e-09 0 0;-1.83e-05 -1.95127744120703e-09 0 0;-1.825e-05 -1.95132614349754e-09 0 0;-1.82e-05 -1.95137484509473e-09 0 0;-1.815e-05 -1.95142354599859e-09 0 0;-1.81e-05 -1.95147224620909e-09 0 0;-1.805e-05 -1.95152094572622e-09 0 0;-1.8e-05 -1.95156964454997e-09 0 0;-1.795e-05 -1.95161834268032e-09 0 0;-1.79e-05 -1.95166704011724e-09 0 0;-1.785e-05 -1.95171573686072e-09 0 0;-1.78e-05 -1.95176443291075e-09 0 0;-1.775e-05 -1.95181312826731e-09 0 0;-1.77e-05 -1.95186182293037e-09 0 0;-1.765e-05 -1.95191051689993e-09 0 0;-1.76e-05 -1.95195921017596e-09 0 0;-1.755e-05 -1.95200790275845e-09 0 0;-1.75e-05 -1.95205659464738e-09 0 0;-1.745e-05 -1.95210528584273e-09 0 0;-1.74e-05 -1.95215397634449e-09 0 0;-1.735e-05 -1.95220266615264e-09 0 0;-1.73e-05 -1.95225135526715e-09 0 0;-1.725e-05 -1.95230004368803e-09 -3503.14903712201 -24106.2645105256;-1.72e-05 -1.95234873141523e-09 -3502.69464411914 -24106.3305390467;-1.715e-05 -1.95239741844876e-09 -3502.24024987174 -24106.3965590027;-1.71e-05 -1.95244610478859e-09 -3501.78585437997 -24106.4625703935;-1.705e-05 -1.95249479043471e-09 -3501.331457644 -24106.5285732191;-1.7e-05 -1.95254347538709e-09 -3500.87705966399 -24106.5945674796;-1.695e-05 -1.95259215964572e-09 -3500.42266044009 -24106.6605531749;-1.69e-05 -1.95264084321058e-09 -3499.96825997248 -24106.7265303049;-1.685e-05 -1.95268952608166e-09 -3499.5138582613 -24106.7924988697;-1.68e-05 -1.95273820825894e-09 -3499.05945530673 -24106.8584588691;-1.675e-05 -1.9527868897424e-09 -3498.60505110892 -24106.9244103033;-1.67e-05 -1.95283557053202e-09 -3498.15064566804 -24106.9903531722;-1.665e-05 -1.95288425062779e-09 -3497.69623898424 -24107.0562874757;-1.66e-05 -1.95293293002969e-09 -3497.2418310577 -24107.1222132138;-1.655e-05 -1.9529816087377e-09 -3496.78742188856 -24107.1881303865;-1.65e-05 -1.9530302867518e-09 -3496.33301147699 -24107.2540389938;-1.645e-05 -1.95307896407199e-09 -3495.87859982316 -24107.3199390357;-1.64e-05 -1.95312764069823e-09 -3495.42418692722 -24107.385830512;-1.635e-05 -1.95317631663051e-09 -3494.96977278933 -24107.4517134229;-1.63e-05 -1.95322499186882e-09 -3494.51535740967 -24107.5175877683;-1.625e-05 -1.95327366641314e-09 -3494.06094078838 -24107.5834535481;-1.62e-05 -1.95332234026344e-09 -3493.60652292563 -24107.6493107624;-1.615e-05 -1.95337101341972e-09 -3493.15210382159 -24107.7151594111;-1.61e-05 -1.95341968588196e-09 -3492.6976834764 -24107.7809994942;-1.605e-05 -1.95346835765013e-09 -3492.24326189024 -24107.8468310116 ...(+21566 chars)]  x2=[-2.04e-05 -1.95027193400208e-09 0 0;-2.035e-05 -1.95032034409549e-09 0 0;-2.03e-05 -1.95036875349594e-09 0 0;-2.025e-05 -1.95041716220342e-09 0 0;-2.02e-05 -1.9504655702179e-09 0 0;-2.015e-05 -1.95051397753937e-09 0 0;-2.01e-05 -1.95056238416782e-09 0 0;-2.005e-05 -1.95061079010321e-09 0 0;-2e-05 -1.95065919534554e-09 0 0;-1.995e-05 -1.9507075998948e-09 0 0;-1.99e-05 -1.95075600375095e-09 0 0;-1.985e-05 -1.95080440691399e-09 0 0;-1.98e-05 -1.9508528093839e-09 0 0;-1.975e-05 -1.95090121116066e-09 0 0;-1.97e-05 -1.95094961224425e-09 0 0;-1.965e-05 -1.95099801263466e-09 0 0;-1.96e-05 -1.95104641233186e-09 0 0;-1.955e-05 -1.95109481133585e-09 0 0;-1.95e-05 -1.95114320964661e-09 0 0;-1.945e-05 -1.95119160726411e-09 0 0;-1.94e-05 -1.95124000418834e-09 0 0;-1.935e-05 -1.95128840041929e-09 0 0;-1.93e-05 -1.95133679595693e-09 0 0;-1.925e-05 -1.95138519080125e-09 0 0;-1.92e-05 -1.95143358495223e-09 0 0;-1.915e-05 -1.95148197840986e-09 0 0;-1.91e-05 -1.95153037117411e-09 0 0;-1.905e-05 -1.95157876324497e-09 0 0;-1.9e-05 -1.95162715462243e-09 0 0;-1.895e-05 -1.95167554530646e-09 0 0;-1.89e-05 -1.95172393529705e-09 0 0;-1.885e-05 -1.95177232459418e-09 0 0;-1.88e-05 -1.95182071319784e-09 0 0;-1.875e-05 -1.951869101108e-09 0 0;-1.87e-05 -1.95191748832465e-09 0 0;-1.865e-05 -1.95196587484778e-09 0 0;-1.86e-05 -1.95201426067736e-09 0 0;-1.855e-05 -1.95206264581338e-09 0 0;-1.85e-05 -1.95211103025582e-09 0 0;-1.845e-05 -1.95215941400466e-09 0 0;-1.84e-05 -1.95220779705989e-09 0 0;-1.835e-05 -1.95225617942149e-09 0 0;-1.83e-05 -1.95230456108944e-09 0 0;-1.825e-05 -1.95235294206372e-09 0 0;-1.82e-05 -1.95240132234433e-09 0 0;-1.815e-05 -1.95244970193123e-09 0 0;-1.81e-05 -1.95249808082442e-09 0 0;-1.805e-05 -1.95254645902387e-09 0 0;-1.8e-05 -1.95259483652957e-09 0 0;-1.795e-05 -1.95264321334151e-09 0 0;-1.79e-05 -1.95269158945966e-09 0 0;-1.785e-05 -1.952739964884e-09 0 0;-1.78e-05 -1.95278833961453e-09 0 0;-1.775e-05 -1.95283671365122e-09 0 0;-1.77e-05 -1.95288508699405e-09 0 0;-1.765e-05 -1.95293345964302e-09 0 0;-1.76e-05 -1.95298183159809e-09 0 0;-1.755e-05 -1.95303020285926e-09 0 0;-1.75e-05 -1.95307857342651e-09 0 0;-1.745e-05 -1.95312694329982e-09 0 0;-1.74e-05 -1.95317531247917e-09 0 0;-1.735e-05 -1.95322368096454e-09 0 0;-1.73e-05 -1.95327204875593e-09 0 0;-1.725e-05 -1.9533204158533e-09 -3502.50631980004 -24104.9633825948;-1.72e-05 -1.95336878225665e-09 -3502.05195132288 -24105.0293990012;-1.715e-05 -1.95341714796596e-09 -3501.59758160143 -24105.0954068429;-1.71e-05 -1.9534655129812e-09 -3501.14321063583 -24105.16140612;-1.705e-05 -1.95351387730237e-09 -3500.68883842627 -24105.2273968323;-1.7e-05 -1.95356224092944e-09 -3500.23446497288 -24105.2933789799;-1.695e-05 -1.9536106038624e-09 -3499.78009027585 -24105.3593525628;-1.69e-05 -1.95365896610124e-09 -3499.32571433532 -24105.4253175809;-1.685e-05 -1.95370732764592e-09 -3498.87133715146 -24105.4912740342;-1.68e-05 -1.95375568849644e-09 -3498.41695872443 -24105.5572219227;-1.675e-05 -1.95380404865279e-09 -3497.96257905439 -24105.6231612463;-1.67e-05 -1.95385240811493e-09 -3497.50819814151 -24105.6890920051;-1.665e-05 -1.95390076688286e-09 -3497.05381598594 -24105.755014199;-1.66e-05 -1.95394912495656e-09 -3496.59943258785 -24105.820927828;-1.655e-05 -1.953997482336e-09 -3496.1450479474 -24105.886832892;-1.65e-05 -1.95404583902118e-09 -3495.69066206475 -24105.9527293911;-1.645e-05 -1.95409419501208e-09 -3495.23627494005 -24106.0186173252;-1.64e-05 -1.95414255030868e-09 -3494.78188657348 -24106.0844966942;-1.635e-05 -1.95419090491095e-09 -3494.3274969652 -24106.1503674983;-1.63e-05 -1.9542392588189e-09 -3493.87310611536 -24106.2162297373;-1.625e-05 -1.95428761203249e-09 -3493.41871402412 -24106.2820834112;-1.62e-05 -1.95433596455171e-09 -3492.96432069166 -24106.34792852;-1.615e-05 -1.95438431637654e-09 -3492.50992611812 -24106.4137650637;-1.61e-05 -1.95443266750697e-09 -3492.05553030368 -24106.4795930423;-1.605e-05 -1.95448101794298e-09 -3491.60113324848 -24106.5454124557;-1.6e-05 ...(+21540 chars)]  x3=[-2.04e-05 -6.84898316736291e-12 0 0;-2.035e-05 -6.84906833275368e-12 0 0;-2.03e-05 -6.84915349571093e-12 0 0;-2.025e-05 -6.84923865623463e-12 0 0;-2.02e-05 -6.84932381432477e-12 0 0;-2.015e-05 -6.8494089699813e-12 0 0;-2.01e-05 -6.84949412320419e-12 0 0;-2.005e-05 -6.84957927399342e-12 0 0;-2e-05 -6.84966442234896e-12 0 0;-1.995e-05 -6.84974956827077e-12 0 0;-1.99e-05 -6.84983471175882e-12 0 0;-1.985e-05 -6.84991985281309e-12 0 0;-1.98e-05 -6.85000499143354e-12 0 0;-1.975e-05 -6.85009012762015e-12 0 0;-1.97e-05 -6.85017526137288e-12 0 0;-1.965e-05 -6.85026039269171e-12 0 0;-1.96e-05 -6.85034552157659e-12 0 0;-1.955e-05 -6.85043064802751e-12 0 0;-1.95e-05 -6.85051577204443e-12 0 0;-1.945e-05 -6.85060089362733e-12 0 0;-1.94e-05 -6.85068601277616e-12 0 0;-1.935e-05 -6.85077112949091e-12 0 0;-1.93e-05 -6.85085624377154e-12 0 0;-1.925e-05 -6.85094135561802e-12 0 0;-1.92e-05 -6.85102646503032e-12 0 0;-1.915e-05 -6.85111157200842e-12 0 0;-1.91e-05 -6.85119667655227e-12 0 0;-1.905e-05 -6.85128177866185e-12 0 0;-1.9e-05 -6.85136687833714e-12 0 0;-1.895e-05 -6.85145197557809e-12 0 0;-1.89e-05 -6.85153707038469e-12 0 0;-1.885e-05 -6.85162216275689e-12 0 0;-1.88e-05 -6.85170725269467e-12 0 0;-1.875e-05 -6.851792340198e-12 0 0;-1.87e-05 -6.85187742526685e-12 0 0;-1.865e-05 -6.85196250790119e-12 0 0;-1.86e-05 -6.85204758810099e-12 0 0;-1.855e-05 -6.85213266586621e-12 0 0;-1.85e-05 -6.85221774119683e-12 0 0;-1.845e-05 -6.85230281409282e-12 0 0;-1.84e-05 -6.85238788455415e-12 0 0;-1.835e-05 -6.85247295258079e-12 0 0;-1.83e-05 -6.8525580181727e-12 0 0;-1.825e-05 -6.85264308132985e-12 0 0;-1.82e-05 -6.85272814205223e-12 0 0;-1.815e-05 -6.85281320033979e-12 0 0;-1.81e-05 -6.85289825619251e-12 0 0;-1.805e-05 -6.85298330961035e-12 0 0;-1.8e-05 -6.85306836059329e-12 0 0;-1.795e-05 -6.85315340914129e-12 0 0;-1.79e-05 -6.85323845525433e-12 0 0;-1.785e-05 -6.85332349893237e-12 0 0;-1.78e-05 -6.85340854017539e-12 0 0;-1.775e-05 -6.85349357898335e-12 0 0;-1.77e-05 -6.85357861535623e-12 0 0;-1.765e-05 -6.85366364929399e-12 0 0;-1.76e-05 -6.85374868079661e-12 0 0;-1.755e-05 -6.85383370986405e-12 0 0;-1.75e-05 -6.85391873649628e-12 0 0;-1.745e-05 -6.85400376069327e-12 0 0;-1.74e-05 -6.854088782455e-12 0 0;-1.735e-05 -6.85417380178143e-12 0 0;-1.73e-05 -6.85425881867253e-12 0 0;-1.725e-05 -6.85434383312828e-12 -11.0557611765581 -79.1592926264141;-1.72e-05 -6.85442884514864e-12 -11.0542690570678 -79.1595010085031;-1.715e-05 -6.85451385473358e-12 -11.0527769336499 -79.1597093624662;-1.71e-05 -6.85459886188307e-12 -11.0512848063048 -79.1599176883034;-1.705e-05 -6.85468386659708e-12 -11.0497926750332 -79.1601259860147;-1.7e-05 -6.85476886887559e-12 -11.0483005398355 -79.1603342555999;-1.695e-05 -6.85485386871855e-12 -11.0468084007122 -79.160542497059;-1.69e-05 -6.85493886612595e-12 -11.045316257664 -79.1607507103919;-1.685e-05 -6.85502386109775e-12 -11.0438241106913 -79.1609588955985;-1.68e-05 -6.85510885363392e-12 -11.0423319597947 -79.1611670526787;-1.675e-05 -6.85519384373442e-12 -11.0408398049747 -79.1613751816326;-1.67e-05 -6.85527883139924e-12 -11.0393476462318 -79.1615832824599;-1.665e-05 -6.85536381662834e-12 -11.0378554835666 -79.1617913551607;-1.66e-05 -6.85544879942169e-12 -11.0363633169795 -79.1619993997349;-1.655e-05 -6.85553377977926e-12 -11.0348711464712 -79.1622074161823;-1.65e-05 -6.85561875770101e-12 -11.0333789720421 -79.1624154045029;-1.645e-05 -6.85570373318693e-12 -11.0318867936927 -79.1626233646967;-1.64e-05 -6.85578870623698e-12 -11.0303946114237 -79.1628312967636;-1.635e-05 -6.85587367685112e-12 -11.0289024252356 -79.1630392007034;-1.63e-05 -6.85595864502933e-12 -11.0274102351288 -79.1632470765162;-1.625e-05 -6.85604361077158e-12 -11.0259180411039 -79.1634549242018;-1.62e-05 -6.85612857407784e-12 -11.0244258431614 -79.1636627437601;-1.615e-05 -6.85621353494808e-12 -11.0229336413019 -79.1638705351912;-1.61e-05 -6.85629849338227e-12 -11.0214414355258 -79.1640782984949;-1.605e-05 -6.85638344938037e-12 -11.0199492258338 -79.1642860336711 ...(+21538 chars)]  x4=[-2.04e-05 4.90518319177223e-13 0 0;-2.035e-05 4.90429267044033e-13 0 0;-2.03e-05 4.9034021473659e-13 0 0;-2.025e-05 4.90251162254927e-13 0 0;-2.02e-05 4.90162109599075e-13 0 0;-2.015e-05 4.90073056769065e-13 0 0;-2.01e-05 4.8998400376493e-13 0 0;-2.005e-05 4.898949505867e-13 0 0;-2e-05 4.89805897234408e-13 0 0;-1.995e-05 4.89716843708085e-13 0 0;-1.99e-05 4.89627790007763e-13 0 0;-1.985e-05 4.89538736133473e-13 0 0;-1.98e-05 4.89449682085247e-13 0 0;-1.975e-05 4.89360627863117e-13 0 0;-1.97e-05 4.89271573467115e-13 0 0;-1.965e-05 4.89182518897271e-13 0 0;-1.96e-05 4.89093464153618e-13 0 0;-1.955e-05 4.89004409236187e-13 0 0;-1.95e-05 4.8891535414501e-13 0 0;-1.945e-05 4.88826298880119e-13 0 0;-1.94e-05 4.88737243441545e-13 0 0;-1.935e-05 4.8864818782932e-13 0 0;-1.93e-05 4.88559132043475e-13 0 0;-1.925e-05 4.88470076084043e-13 0 0;-1.92e-05 4.88381019951054e-13 0 0;-1.915e-05 4.8829196364454e-13 0 0;-1.91e-05 4.88202907164534e-13 0 0;-1.905e-05 4.88113850511066e-13 0 0;-1.9e-05 4.88024793684169e-13 0 0;-1.895e-05 4.87935736683874e-13 0 0;-1.89e-05 4.87846679510212e-13 0 0;-1.885e-05 4.87757622163216e-13 0 0;-1.88e-05 4.87668564642916e-13 0 0;-1.875e-05 4.87579506949345e-13 0 0;-1.87e-05 4.87490449082534e-13 0 0;-1.865e-05 4.87401391042515e-13 0 0;-1.86e-05 4.8731233282932e-13 0 0;-1.855e-05 4.87223274442979e-13 0 0;-1.85e-05 4.87134215883526e-13 0 0;-1.845e-05 4.87045157150991e-13 0 0;-1.84e-05 4.86956098245405e-13 0 0;-1.835e-05 4.86867039166802e-13 0 0;-1.83e-05 4.86777979915212e-13 0 0;-1.825e-05 4.86688920490667e-13 0 0;-1.82e-05 4.86599860893198e-13 0 0;-1.815e-05 4.86510801122838e-13 0 0;-1.81e-05 4.86421741179618e-13 0 0;-1.805e-05 4.86332681063569e-13 0 0;-1.8e-05 4.86243620774723e-13 0 0;-1.795e-05 4.86154560313113e-13 0 0;-1.79e-05 4.86065499678768e-13 0 0;-1.785e-05 4.85976438871722e-13 0 0;-1.78e-05 4.85887377892006e-13 0 0;-1.775e-05 4.85798316739651e-13 0 0;-1.77e-05 4.85709255414689e-13 0 0;-1.765e-05 4.85620193917152e-13 0 0;-1.76e-05 4.85531132247071e-13 0 0;-1.755e-05 4.85442070404478e-13 0 0;-1.75e-05 4.85353008389405e-13 0 0;-1.745e-05 4.85263946201883e-13 0 0;-1.74e-05 4.85174883841944e-13 0 0;-1.735e-05 4.8508582130962e-13 0 0;-1.73e-05 4.84996758604942e-13 0 0;-1.725e-05 4.84907695727941e-13 -12.4386859981126 -78.9096038524822;-1.72e-05 4.8481863267865e-13 -12.4371985849279 -78.9098383022075;-1.715e-05 4.84729569457101e-13 -12.4357111673243 -78.9100727238956;-1.71e-05 4.84640506063324e-13 -12.4342237453021 -78.9103071175466;-1.705e-05 4.84551442497351e-13 -12.432736318862 -78.9105414831602;-1.7e-05 4.84462378759215e-13 -12.4312488880044 -78.9107758207365;-1.695e-05 4.84373314848946e-13 -12.42976145273 -78.9110101302753;-1.69e-05 4.84284250766577e-13 -12.4282740130392 -78.9112444117766;-1.685e-05 4.84195186512139e-13 -12.4267865689325 -78.9114786652403;-1.68e-05 4.84106122085663e-13 -12.4252991204106 -78.9117128906662;-1.675e-05 4.84017057487182e-13 -12.4238116674739 -78.9119470880544;-1.67e-05 4.83927992716727e-13 -12.4223242101229 -78.9121812574047;-1.665e-05 4.83838927774329e-13 -12.4208367483582 -78.9124153987171;-1.66e-05 4.8374986266002e-13 -12.4193492821803 -78.9126495119914;-1.655e-05 4.83660797373833e-13 -12.4178618115897 -78.9128835972276;-1.65e-05 4.83571731915798e-13 -12.416374336587 -78.9131176544256;-1.645e-05 4.83482666285947e-13 -12.4148868571727 -78.9133516835853;-1.64e-05 4.83393600484312e-13 -12.4133993733473 -78.9135856847066;-1.635e-05 4.83304534510924e-13 -12.4119118851114 -78.9138196577895;-1.63e-05 4.83215468365815e-13 -12.4104243924654 -78.9140536028339;-1.625e-05 4.83126402049018e-13 -12.4089368954099 -78.9142875198396;-1.62e-05 4.83037335560562e-13 -12.4074493939455 -78.9145214088067;-1.615e-05 4.82948268900481e-13 -12.4059618880726 -78.9147552697349;-1.61e-05 4.82859202068806e-13 -12.4044743777919 -78.9149891026243;-1.605e-05 4.82770135065567e-13 -12.4029868631037 -78.9152229074748;-1.6e-05 4.82681067890798e-13 -12.4014993440087 -78.9154566842862;-1.595e-05 ...(+21165 chars)]  x5=2.03919101606495e-05  V1=[0 0 0 2.827e-09 2.436e+04 2.436e+04;0 0 0 377 377 377;1.571 1.571 1.571 -0.5179 -0.1443 -1.715]  V2=[0 0 0 2.868e-09 2.436e+04 2.436e+04;0 0 0 377 377 377;1.571 1.571 1.571 -0.5251 -0.1443 -1.715]  I1=[0 0 0 7.018e-12 79.92 79.92;0 0 0 377 377 377;1.571 1.571 1.571 -1.622 -0.1386 -1.709]  I2=[0 0 0 7.946e-12 79.89 79.89;0 0 0 377 377 377;1.571 1.571 1.571 0.3547 -0.1565 -1.727]  nHarmo=2  Measurements=None  Decoupling=off  VsMag0=0  VrMag0=0  VsAngle0=0  VrAngle0=0  IsMag0=0  IrMag0=0  IsAngle0=0  IrAngle0=0
  Ground3 : spsGroundLib/Ground  LConnTagsString=a
  "Grounding Transformer " : spsGroundingTransformerLib/Grounding Transformer   UNITS=pu  NominalPower="[100e6   60]"  NominalVoltage=25e3  ZeroSequenceImpedance_pu=[0.025 0.75]  MagnetizationBranch_pu=[500 500]  ZeroSequenceImpedance_SI=[0.052083 589.05]  MagnetizationBranch_SI=[1041.7 3.927e+005]  Measurements=None
  A : PMIOPort  Side=Left
  B : PMIOPort  Port=2  Side=Left
  C : PMIOPort  Port=3  Side=Left
  connections:
  "3.3ohms "/RConn1 -- Ground3/LConn1
  120 kV / 25 kV 47 MVA/LConn1 -- 120kV 2500MVA/RConn1
  120 kV / 25 kV 47 MVA/LConn2 -- 120kV 2500MVA/RConn2
  120 kV / 25 kV 47 MVA/LConn3 -- 120kV 2500MVA/RConn3
  120 kV / 25 kV 47 MVA/RConn1 -- "Grounding Transformer "/LConn1 -- 14-km Feeder/RConn1 -- 30-MW 2-Mvar Load/LConn1
  120 kV / 25 kV 47 MVA/RConn2 -- "Grounding Transformer "/LConn2 -- 14-km Feeder/RConn2 -- 30-MW 2-Mvar Load/LConn2
  120 kV / 25 kV 47 MVA/RConn3 -- "Grounding Transformer "/LConn3 -- 14-km Feeder/RConn3 -- 30-MW 2-Mvar Load/LConn3
  5-km Feeder/RConn1 -- 14-km Feeder/LConn1 -- 2-MW Load/LConn1
  5-km Feeder/RConn2 -- 14-km Feeder/LConn2 -- 2-MW Load/LConn2
  5-km Feeder/RConn3 -- 14-km Feeder/LConn3 -- 2-MW Load/LConn3
  A/RConn1 -- 5-km Feeder/LConn1
  B/RConn1 -- 5-km Feeder/LConn2
  C/RConn1 -- 5-km Feeder/LConn3
  "Grounding Transformer "/RConn1 -- "3.3ohms "/LConn1
